simulink model "ex5p3"  (R2016b)
settings: Solver=VariableStepAuto  StartTime=0.0  StopTime=1  RelTol=1e-3
undefined symbols (not defined in the file): alpha
libraries: powerlib x10, simulink x6, powerlib_meascontrol x3
settings Model: Creator=user  LastModifiedBy=user

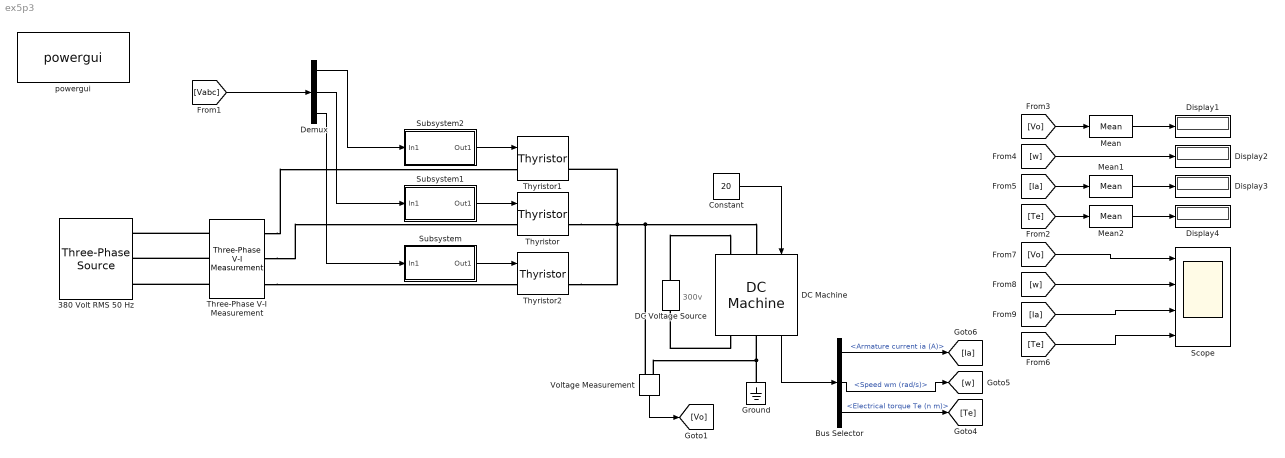
== system ex5p3 ==
  note: 300v
  380 Volt RMS 50 Hz : powerlib/Electrical Sources/Three-Phase Source  InternalConnection=Yg  VoltagePhases=off  Voltage=380  PhaseAngle=0  Voltage_phases=[25e3 25e3 25e3]/sqrt(3)  PhaseAngles_phases=[0 -120 +120]  Frequency=50  NonIdealSource=off  SpecifyImpedance=off  Resistance=0.8929  Inductance=16.58e-3  ShortCircuitLevel=100e6  BaseVoltage=25e3  XRratio=7  BusType=swing  Pref=10e3  Qref=0  Prefabc=[10e3, 10e3, 10e3]  Qrefabc=[0, 0, 0]  Qmin=-inf  Qmax=inf
  Bus Selector : BusSelector  OutputSignals=Armature current ia (A),Speed wm (rad/s),Electrical torque Te (n m)
  Constant : Constant  Value=20
  DC Machine : powerlib/Machines/DC Machine  PresetModel=01: 5HP 240V 1750RPM Field:300V  MechanicalLoad=Torque TL  FieldType=Wound  ShowDetailedParameters=on  MeasurementBus=off  RLa=[2.581 0.028]  RLf=[281.3 156]  Laf=0.9483  MachineConstant=Torque constant (N.m/A)  Ke=1.8  Kt=1.8  J=0.02215  Bm=0.002953  Tf=0.5161  w0=1  Ifinit=1  TsPowergui=0  TsBlock=-1
  DC Voltage Source : powerlib/Electrical Sources/DC Voltage Source  Amplitude=300  Measurements=None
  Demux : Demux  Outputs=3
  Display{1..4} (4 alike) : Display
  Ground : powerlib/Elements/Ground  LConnTagsString=a
  Mean : powerlib_meascontrol/Measurements/Mean  Freq=50  Vinit=0  Ts=0
  Mean1 : powerlib_meascontrol/Measurements/Mean  Freq=50  Vinit=0  Ts=0
  Mean2 : powerlib_meascontrol/Measurements/Mean  Freq=50  Vinit=0  Ts=0
  Scope : Scope  NumInputPorts=4
  Subsystem : Subsystem
  Subsystem1 : Subsystem
  Subsystem2 : Subsystem
  Three-Phase V-I Measurement : powerlib/Measurements/Three-Phase V-I Measurement  VoltageMeasurement=phase-to-ground  SetLabelV=on  LabelV=Vabc  Vpu=off  VpuLL=off  CurrentMeasurement=yes  SetLabelI=on  LabelI=Iabc  Ipu=off  Pbase=100e6  Vbase=500e3  OutputType=Complex  PhasorSimulation=off  PSBequivalent=0
  Thyristor : powerlib/Power Electronics/Thyristor  Ron=0.001  Lon=0  Vf=0.8  IC=0  Rs=500  Cs=250e-9  Measurements=on
  Thyristor1 : powerlib/Power Electronics/Thyristor  Ron=0.001  Lon=0  Vf=0.8  IC=0  Rs=500  Cs=250e-9  Measurements=on
  Thyristor2 : powerlib/Power Electronics/Thyristor  Ron=0.001  Lon=0  Vf=0.8  IC=0  Rs=500  Cs=250e-9  Measurements=on
  Voltage Measurement : powerlib/Measurements/Voltage Measurement  PhasorSimulation=off  OutputType=Complex  PSBequivalent=0
  powergui : powerlib/powergui  Priority=1  SimulationMode=Discrete  SolverType=Tustin/Backward Euler (TBE)  SampleTime=5e-6  frequency=60  SPID=off  DisableSnubberDevices=off  DisableRonSwitches=off  DisableVfSwitches=off  SwTol=0  DisplayEquations=off  Interpol=off  ExternalGateDelay=off  methode=off  Ts=10  FunctionMessages=off  echomessages=off  HookPort=off  EnableUseOfTLC=off  x0status=blocks  frequencyindice=50  Pbase=100e6  ErrMax=1e-4  Iterations=50  UnitsV=kV  UnitsW=MW  buscounter=0  RestoreLinks=warning  ResistiveCurrentMeasurement=off  Frange=[0:2:500]  Ylog=off  Xlog=on  ShowGrid=off  save=off  variable=ZData  structure=0  ZoomFFT=off  StartTime=0.0  cycles=1  DisplayStyle=1  fundamental=60  FreqAxis=off  MaxFrequency=1000  frequencyindicesteady=1  RmsSteady=1  display=off
  wires:
  Subsystem2/1(Out1) -> Thyristor1/1
  Subsystem1/1(Out1) -> Thyristor/1
  Subsystem/1(Out1) -> Thyristor2/1
  [Vabc] -> Demux/1
  Demux/2 -> Subsystem1/1(In1)
  Demux/1 -> Subsystem2/1(In1)
  Demux/3 -> Subsystem/1(In1)
  [Vo] -> Mean/1
  Constant/1 -> DC Machine/1
  Voltage Measurement/1 -> [Vo]
  DC Machine/1 -> Bus Selector/1
  Bus Selector/1 -> [Ia]  "<Armature current ia (A)>"
  Bus Selector/2 -> [w]  "<Speed wm (rad/s)>"
  Bus Selector/3 -> [Te]  "<Electrical torque Te (n m)>"
  Mean/1 -> Display1/1
  [w] -> Display2/1
  [Ia] -> Mean1/1
  Mean1/1 -> Display3/1
  [Te] -> Mean2/1
  Mean2/1 -> Display4/1
  [Vo] -> Scope/1
  [w] -> Scope/2
  [Ia] -> Scope/3
  [Te] -> Scope/4
  connections:
  Thyristor2/RConn1 -- Voltage Measurement/LConn1 -- DC Machine/LConn1 -- Thyristor1/RConn1 -- Thyristor/RConn1
  Three-Phase V-I Measurement/RConn3 -- Thyristor2/LConn1
  Three-Phase V-I Measurement/LConn3 -- 380 Volt RMS 50 Hz/RConn3
  Three-Phase V-I Measurement/LConn2 -- 380 Volt RMS 50 Hz/RConn2
  Three-Phase V-I Measurement/RConn2 -- Thyristor/LConn1
  Three-Phase V-I Measurement/RConn1 -- Thyristor1/LConn1
  Three-Phase V-I Measurement/LConn1 -- 380 Volt RMS 50 Hz/RConn1
  DC Voltage Source/RConn1 -- DC Machine/LConn2
  DC Machine/RConn2 -- DC Voltage Source/LConn1
  Voltage Measurement/LConn2 -- DC Machine/RConn1 -- Ground/LConn1

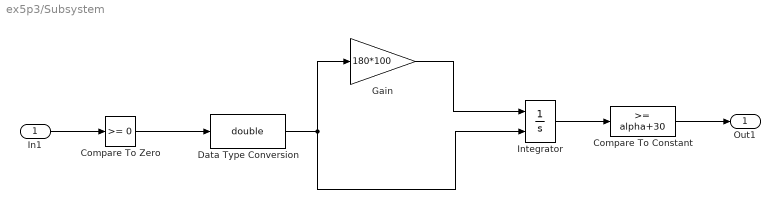
== system ex5p3/Subsystem ==
  In1 : Inport
  Compare To Constant : simulink/Logic and Bit Operations/Compare To Constant  relop=>=  const=alpha+30  OutDataTypeStr=boolean
  Compare To Zero : simulink/Logic and Bit Operations/Compare To Zero  relop=>=  OutDataTypeStr=boolean
  Data Type Conversion : DataTypeConversion  OutDataTypeStr=double
  Gain : Gain  Gain=180*100
  Integrator : Integrator  ExternalReset=falling
  Out1 : Outport
  wires:
  Data Type Conversion/1 -> Gain/1, Integrator/2
  Compare To Constant/1 -> Out1/1
  In1/1 -> Compare To Zero/1
  Integrator/1 -> Compare To Constant/1
  Compare To Zero/1 -> Data Type Conversion/1
  Gain/1 -> Integrator/1

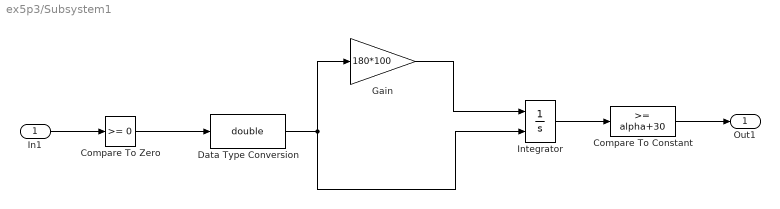
== system ex5p3/Subsystem1 ==
  In1 : Inport
  Compare To Constant : simulink/Logic and Bit Operations/Compare To Constant  relop=>=  const=alpha+30  OutDataTypeStr=boolean
  Compare To Zero : simulink/Logic and Bit Operations/Compare To Zero  relop=>=  OutDataTypeStr=boolean
  Data Type Conversion : DataTypeConversion  OutDataTypeStr=double
  Gain : Gain  Gain=180*100
  Integrator : Integrator  ExternalReset=falling
  Out1 : Outport
  wires:
  Data Type Conversion/1 -> Gain/1, Integrator/2
  Compare To Constant/1 -> Out1/1
  In1/1 -> Compare To Zero/1
  Integrator/1 -> Compare To Constant/1
  Compare To Zero/1 -> Data Type Conversion/1
  Gain/1 -> Integrator/1

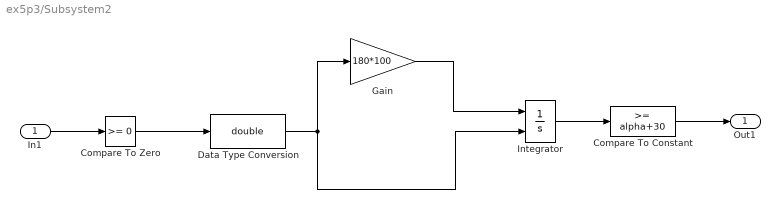
== system ex5p3/Subsystem2 ==
  In1 : Inport
  Compare To Constant : simulink/Logic and Bit Operations/Compare To Constant  relop=>=  const=alpha+30  OutDataTypeStr=boolean
  Compare To Zero : simulink/Logic and Bit Operations/Compare To Zero  relop=>=  OutDataTypeStr=boolean
  Data Type Conversion : DataTypeConversion  OutDataTypeStr=double
  Gain : Gain  Gain=180*100
  Integrator : Integrator  ExternalReset=falling
  Out1 : Outport
  wires:
  Data Type Conversion/1 -> Gain/1, Integrator/2
  Compare To Constant/1 -> Out1/1
  In1/1 -> Compare To Zero/1
  Integrator/1 -> Compare To Constant/1
  Compare To Zero/1 -> Data Type Conversion/1
  Gain/1 -> Integrator/1
